simulink model "PID_Control_Soln"  (R2024a)
settings: Solver=VariableStepAuto  StartTime=0.0  StopTime=10.0  RelTol=1e-3
settings Model: Creator=nroberts  LastModifiedBy=nroberts

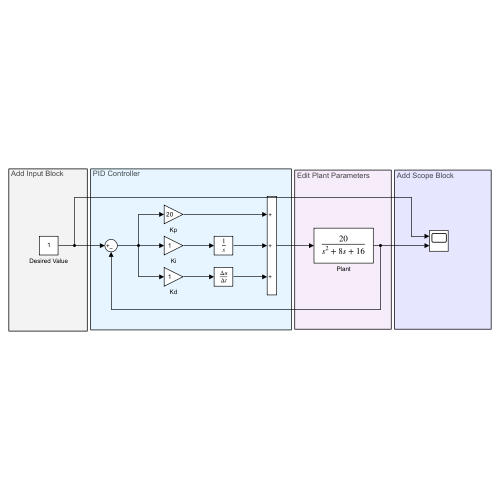
[thumbnail: Simulink's stored preview of the top-level diagram]
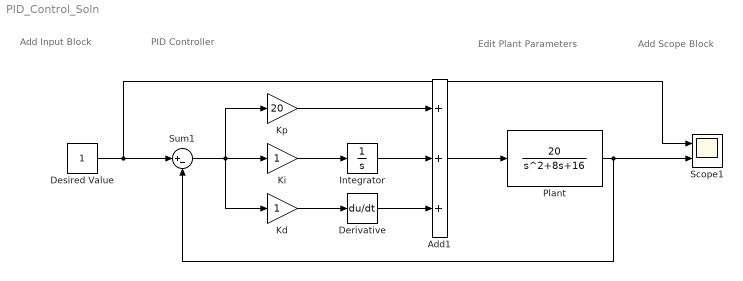
== system PID_Control_Soln ==
  note: Edit Plant Parameters
  note: PID Controller
  note: Add Input Block
  note: Add Scope Block
  Add1 : Sum  Inputs=+++
  Derivative : Derivative
  Desired Value : Constant
  Integrator : Integrator
  Kd : Gain
  Ki : Gain
  Kp : Gain  Gain=20
  Plant : TransferFcn  Numerator=[20]  Denominator=[1 8 16]
  Scope1 : Scope  NumInputPorts=2
  Sum1 : Sum  Inputs=|+-
  wires:
  Add1/1 -> Plant/1
  Plant/1 -> Sum1/2, Scope1/2
  Derivative/1 -> Add1/3
  Kd/1 -> Derivative/1
  Sum1/1 -> Kp/1, Kd/1, Ki/1
  Integrator/1 -> Add1/2
  Ki/1 -> Integrator/1
  Desired Value/1 -> Sum1/1, Scope1/1
  Kp/1 -> Add1/1
